simulink library "Enrg_conv_El_to_Mec_zfCetrax"  (R2016a)
settings: Solver=ode1  StartTime=0.0  StopTime=Inf  FixedStep=0.001  RelTol=1e-3
undefined symbols (not defined in the file): drvEmot_RefTqeMOT, FirstDrivenAxle_FirstDrivenAxleNoOfEmot, FirstDrivenAxleNoOfEmot, FMIKit, mec_fRollCoeffOverall, mec_iDiffAxle, mec_massVehicle_kg, mec_rWheelDriven, RefTqeMOT, SecondDrivenAxle_SecondDrivenAxleNoOfEmot, SecondDrivenAxleNoOfEmot
libraries: simulink_extras x3, Enrg_conv_El_to_Mec_zfCetrax x3
(part 1 of 3)
settings Model: Creator=SAHOPRA  LastModifiedBy=KGNANPR
settings DataIOCC: LimitDataPoints=on  SaveFormat=Array
settings OptimizationCC: BlockReduction=off  OptimizeBlockIOStorage=off  BufferReuse=off  GlobalBufferReuse=off  ExpressionFolding=off  ExpressionDepthLimit=2147483647  LocalBlockOutputs=off
settings DebuggingCC: UnderspecifiedInitializationDetection=Classic  MergeDetectMultiDrivingBlocksExec=none  SolverPrmCheckMsg=warning  StateNameClashWarn=warning
settings HardwareCC: ProdBitPerPointer=32  ProdLargestAtomicFloat=None  ProdIntDivRoundTo=Undefined  ProdEndianess=Unspecified  ProdWordSize=32  ProdHWDeviceType=32-bit Generic
settings ModelReferenceCC: PropagateSignalLabelsOutOfModel=off
settings SFSimCC: SimUserSources="\"C:\\ORNOVNU\\01_DIVe\\drl_dev_hvlv_work\\ldDevProj\\case\\c000\\Content\\phys\\hvs\\Support\\FMIToolkit\\FMIKit-Simulink-2.9\\src\\FMU.cpp\" \"C:\\ORNOVNU\\01_DIVe\\drl_dev_hvlv_work\\ldDevProj\\case\\c000\\Content\\phys\\hvs\\Support\\FMIToolkit\\FMIKit-Simulink-2.9\\src\\FMU1.cpp\" \"C:\\ORNOVNU\\01_DIVe\\drl_dev_hvlv_work\\ldDevProj\\case\\c000\\Content\\phys\\hvs\\Support\\FMIToolkit\\FMIKit-Simulink-2.9\\src\\FMU2.cpp\" \"C:\\ORNOVNU\\01_DIVe\\drm_dev_hvlv_work\\Content\\phys\\hvs\\Support\\FMIToolkit\\FMIKit-Simulink-2.9\\src\\FMU.cpp\" \"C:\\ORNOVNU\\01_DIVe\\drm_dev_hvlv_work\\Content\\phys\\hvs\\Support\\FMIToolkit\\FMIKit-Simulink-2.9\\src\\FMU1.cpp\" \"C:\\ORNOVNU\\01_DIVe\\drm_dev_hvlv_work\\Content\\phys\\hvs\\Support\\FMIToolkit\\FMIKit-Simulink-2.9\\src\\FMU2.cpp\" \"C:\\ORNOVNU\\01_DIVe\\drm_dev_hvlv_work\\Content\\phys\\hvs\\detailed\\Support\\FMIToolkit\\FMIKit-Simulink-2.9\\src\\FMU.cpp\" \"C:\\ORNOVNU\\01_DIVe\\drm_dev_hvlv_work\\Content\\phys\\hvs\\detailed\\Support\\FMIToolkit\\FMIKit-Simulink-2.9\\src\\FMU1.cpp\" \"C:\\ORNOVNU\\01_DIVe\\drm_dev_hvlv_work\\Content\\phys\\hvs\\detailed\\Support\\FMIToolkit\\FMIKit-Simulink-2.9\\src\\FMU2.cpp\" \"Y:\\03_Tasks\\20210223_OrNu_HVSDive_BoschModelle\\02_WIP\\FMIKit-Simulink-2.9\\src\\FMU.cpp\" \"Y:\\03_Tasks\\20210223_OrNu_HVSDive_BoschModelle\\02_WIP\\FMIKit-Simulink-2.9\\src\\FMU1.cpp\" \"Y:\\03_Tasks\\20210223_OrNu_HVSDive_BoschModelle\\02_WIP\\FMIKit-Simulink-2.9\\src\\FMU2.cpp\" \"C:\\Temp_Data\\eBus_work\\Content\\phys\\hvs\\detailed\\Support\\FMIToolkit\\FMIKit-Simulink-2.9\\src\\FMU.cpp\" \"C:\\Temp_Data\\eBus_work\\Content\\phys\\hvs\\detailed\\Support\\FMIToolkit\\FMIKit-Simulink-2.9\\src\\FMU1.cpp\" \"C:\\Temp_Data\\eBus_work\\Content\\phys\\hvs\\detailed\\Support\\FMIToolkit\\FMIKit-Simulink-2.9\\src\\FMU2.cpp\" \"C:\\Temp_Data\\DIVeMB\\00_eBus_Work\\Content\\phys\\hvs\\detailed\\Support\\FMIToolkit\\FMIKit-Simulink-2.9\\src\\FMU.cpp\" \"C:\\Temp_Data\\DIVeMB\\00_eBus_Work\\Content\\phys\\hvs\\detailed\\Support\\FMIToolkit\\FMIKit-Simulink-2.9\\src\\FMU1.cpp\" \"C:\\Temp_Data\\DIVeMB\\00_eBus_Work\\Content\\phys\\hvs\\detailed\\Support\\FMIToolkit\\FMIKit-Simulink-2.9\\src\\FMU2.cpp\" \"C:\\Temp_Data\\DIVeMB\\eBus_work\\Content\\phys\\hvs\\detailed\\Support\\FMIToolkit\\FMIKit-Simulink-2.9\\src\\FMU.cpp\" \"C:\\Temp_Data\\DIVeMB\\eBus_work\\Content\\phys\\hvs\\detailed\\Support\\FMIToolkit\\FMIKit-Simulink-2.9\\src\\FMU1.cpp\" \"C:\\Temp_Data\\DIVeMB\\eBus_work\\Content\\phys\\hvs\\detailed\\Support\\FMIToolkit\\FMIKit-Simulink-2.9\\src\\FMU2.cpp\""  SimUserIncludeDirs="\"C:\\ORNOVNU\\01_DIVe\\drl_dev_hvlv_work\\ldDevProj\\case\\c000\\Content\\phys\\hvs\\Support\\FMIToolkit\\FMIKit-Simulink-2.9\\include\" \"C:\\ORNOVNU\\01_DIVe\\drm_dev_hvlv_work\\Content\\phys\\hvs\\Support\\FMIToolkit\\FMIKit-Simulink-2.9\\include\" \"C:\\ORNOVNU\\01_DIVe\\drm_dev_hvlv_work\\Content\\phys\\hvs\\detailed\\Support\\FMIToolkit\\FMIKit-Simulink-2.9\\include\" \"Y:\\03_Tasks\\20210223_OrNu_HVSDive_BoschModelle\\02_WIP\\FMIKit-Simulink-2.9\\include\" \"C:\\Temp_Data\\eBus_work\\Content\\phys\\hvs\\detailed\\Support\\FMIToolkit\\FMIKit-Simulink-2.9\\include\" \"C:\\Temp_Data\\DIVeMB\\00_eBus_Work\\Content\\phys\\hvs\\detailed\\Support\\FMIToolkit\\FMIKit-Simulink-2.9\\include\" \"C:\\Temp_Data\\DIVeMB\\eBus_work\\Content\\phys\\hvs\\detailed\\Support\\FMIToolkit\\FMIKit-Simulink-2.9\\include\""
settings RTWCC: SystemTargetFile=rti1005.tlc  MakeCommand=make_rti  TemplateMakefile=rti1005.tmf  Description=dSPACE DS1005 Hardware Platform  CustomInclude="\"C:\\ORNOVNU\\01_DIVe\\drl_dev_hvlv_work\\ldDevProj\\case\\c000\\Content\\phys\\hvs\\Support\\FMIToolkit\\FMIKit-Simulink-2.9\\include\" \"C:\\ORNOVNU\\01_DIVe\\drm_dev_hvlv_work\\Content\\phys\\hvs\\Support\\FMIToolkit\\FMIKit-Simulink-2.9\\include\" \"C:\\ORNOVNU\\01_DIVe\\drm_dev_hvlv_work\\Content\\phys\\hvs\\detailed\\Support\\FMIToolkit\\FMIKit-Simulink-2.9\\include\" \"Y:\\03_Tasks\\20210223_OrNu_HVSDive_BoschModelle\\02_WIP\\FMIKit-Simulink-2.9\\include\" \"C:\\Temp_Data\\eBus_work\\Content\\phys\\hvs\\detailed\\Support\\FMIToolkit\\FMIKit-Simulink-2.9\\include\" \"C:\\Temp_Data\\DIVeMB\\00_eBus_Work\\Content\\phys\\hvs\\detailed\\Support\\FMIToolkit\\FMIKit-Simulink-2.9\\include\" \"C:\\Temp_Data\\DIVeMB\\eBus_work\\Content\\phys\\hvs\\detailed\\Support\\FMIToolkit\\FMIKit-Simulink-2.9\\include\""  CustomSource="\"C:\\ORNOVNU\\01_DIVe\\drl_dev_hvlv_work\\ldDevProj\\case\\c000\\Content\\phys\\hvs\\Support\\FMIToolkit\\FMIKit-Simulink-2.9\\src\\FMU.cpp\" \"C:\\ORNOVNU\\01_DIVe\\drl_dev_hvlv_work\\ldDevProj\\case\\c000\\Content\\phys\\hvs\\Support\\FMIToolkit\\FMIKit-Simulink-2.9\\src\\FMU1.cpp\" \"C:\\ORNOVNU\\01_DIVe\\drl_dev_hvlv_work\\ldDevProj\\case\\c000\\Content\\phys\\hvs\\Support\\FMIToolkit\\FMIKit-Simulink-2.9\\src\\FMU2.cpp\" \"C:\\ORNOVNU\\01_DIVe\\drm_dev_hvlv_work\\Content\\phys\\hvs\\Support\\FMIToolkit\\FMIKit-Simulink-2.9\\src\\FMU.cpp\" \"C:\\ORNOVNU\\01_DIVe\\drm_dev_hvlv_work\\Content\\phys\\hvs\\Support\\FMIToolkit\\FMIKit-Simulink-2.9\\src\\FMU1.cpp\" \"C:\\ORNOVNU\\01_DIVe\\drm_dev_hvlv_work\\Content\\phys\\hvs\\Support\\FMIToolkit\\FMIKit-Simulink-2.9\\src\\FMU2.cpp\" \"C:\\ORNOVNU\\01_DIVe\\drm_dev_hvlv_work\\Content\\phys\\hvs\\detailed\\Support\\FMIToolkit\\FMIKit-Simulink-2.9\\src\\FMU.cpp\" \"C:\\ORNOVNU\\01_DIVe\\drm_dev_hvlv_work\\Content\\phys\\hvs\\detailed\\Support\\FMIToolkit\\FMIKit-Simulink-2.9\\src\\FMU1.cpp\" \"C:\\ORNOVNU\\01_DIVe\\drm_dev_hvlv_work\\Content\\phys\\hvs\\detailed\\Support\\FMIToolkit\\FMIKit-Simulink-2.9\\src\\FMU2.cpp\" \"Y:\\03_Tasks\\20210223_OrNu_HVSDive_BoschModelle\\02_WIP\\FMIKit-Simulink-2.9\\src\\FMU.cpp\" \"Y:\\03_Tasks\\20210223_OrNu_HVSDive_BoschModelle\\02_WIP\\FMIKit-Simulink-2.9\\src\\FMU1.cpp\" \"Y:\\03_Tasks\\20210223_OrNu_HVSDive_BoschModelle\\02_WIP\\FMIKit-Simulink-2.9\\src\\FMU2.cpp\" \"C:\\Temp_Data\\eBus_work\\Content\\phys\\hvs\\detailed\\Support\\FMIToolkit\\FMIKit-Simulink-2.9\\src\\FMU.cpp\" \"C:\\Temp_Data\\eBus_work\\Content\\phys\\hvs\\detailed\\Support\\FMIToolkit\\FMIKit-Simulink-2.9\\src\\FMU1.cpp\" \"C:\\Temp_Data\\eBus_work\\Content\\phys\\hvs\\detailed\\Support\\FMIToolkit\\FMIKit-Simulink-2.9\\src\\FMU2.cpp\" \"C:\\Temp_Data\\DIVeMB\\00_eBus_Work\\Content\\phys\\hvs\\detailed\\Support\\FMIToolkit\\FMIKit-Simulink-2.9\\src\\FMU.cpp\" \"C:\\Temp_Data\\DIVeMB\\00_eBus_Work\\Content\\phys\\hvs\\detailed\\Support\\FMIToolkit\\FMIKit-Simulink-2.9\\src\\FMU1.cpp\" \"C:\\Temp_Data\\DIVeMB\\00_eBus_Work\\Content\\phys\\hvs\\detailed\\Support\\FMIToolkit\\FMIKit-Simulink-2.9\\src\\FMU2.cpp\" \"C:\\Temp_Data\\DIVeMB\\eBus_work\\Content\\phys\\hvs\\detailed\\Support\\FMIToolkit\\FMIKit-Simulink-2.9\\src\\FMU.cpp\" \"C:\\Temp_Data\\DIVeMB\\eBus_work\\Content\\phys\\hvs\\detailed\\Support\\FMIToolkit\\FMIKit-Simulink-2.9\\src\\FMU1.cpp\" \"C:\\Temp_Data\\DIVeMB\\eBus_work\\Content\\phys\\hvs\\detailed\\Support\\FMIToolkit\\FMIKit-Simulink-2.9\\src\\FMU2.cpp\""
settings STFCustomTargetCC: ModelReferenceCompliant=off  GeneratePreprocessorConditionals=Disable all  CombineOutputUpdateFcns=on  MatFileLogging=on  CPPClassGenCompliant=on  GRTInterface=off  SystemTargetFile=rti1005.tlc
settings GRTTargetCC: ModelReferenceCompliant=off  ParMdlRefBuildCompliant=off  CompOptLevelCompliant=off  ConcurrentExecutionCompliant=off  UseToolchainInfoCompliant=off
settings ConfigComp: CovModelRefEnable=Off

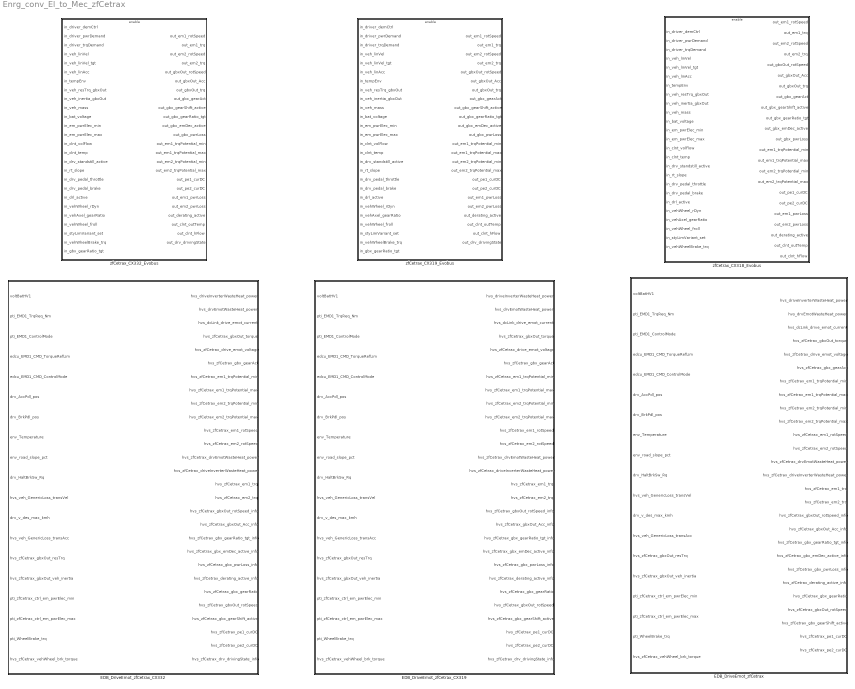
== system Enrg_conv_El_to_Mec_zfCetrax ==
  EDB_DriveEmot_zfCetrax : Subsystem
  EDB_DriveEmot_zfCetrax_CX319 : Subsystem
  EDB_DriveEmot_zfCetrax_CX332 : Subsystem
  zfCetrax_CX318_Evobus : Subsystem  mask(MapModule){}
  zfCetrax_CX319_Evobus : Subsystem  mask(MapModule){}
  zfCetrax_CX332_Evobus : Subsystem  mask(MapModule){}

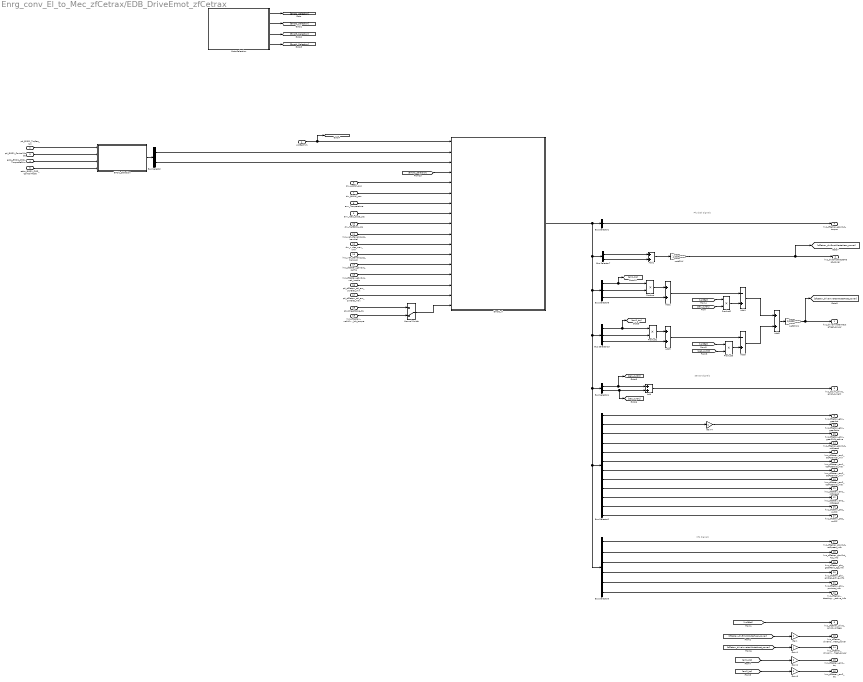
== system Enrg_conv_El_to_Mec_zfCetrax/EDB_DriveEmot_zfCetrax ==
  note: Physical Signals
  note: Sensor Signals
  note: Info Signals
  voltBatHV1 : Inport
  pti_EMD1_TrqReq_Nm : Inport  Port=2
  pti_EMD1_ControlMode : Inport  Port=3
  edcu_EMD1_CMD_TorqueRefLim : Inport  Port=4
  edcu_EMD1_CMD_ControlMode : Inport  Port=5
  drv_AccPdl_pos : Inport  Port=6
  drv_BrkPdl_pos : Inport  Port=7
  env_Temperature : Inport  Port=8
  env_road_slope_pct : Inport  Port=9
  drv_HaltBrkSw_Rq : Inport  Port=10
  hvs_veh_GenericLoss_transVel : Inport  Port=11
  drv_v_des_max_kmh : Inport  Port=12
  hvs_veh_GenericLoss_transAcc : Inport  Port=13
  hvs_zfCetrax_gbxOut_resTrq : Inport  Port=14
  hvs_zfCetrax_gbxOut_veh_inertia : Inport  Port=15
  pti_zfCetrax_ctrl_em_pwrElec_min : Inport  Port=16
  pti_zfCetrax_ctrl_em_pwrElec_max : Inport  Port=17
  pti_WheelBrake_trq : Inport  Port=18
  hvs_zfCetrax_vehWheel_brk_torque : Inport  Port=19
  Add{,1..3,6} (5 alike) : Sum
  Add4 : Sum  Inputs=-+
  Add5 : Sum  Inputs=-+
  Bus Selector : BusSelector  OutputSignals=EMD1_TrqReq_Nm,EMD1_ControlMode
  Bus Selector1 : BusSelector  OutputSignals=gbx_out.gbxOut_trq
  Bus Selector13 : BusSelector  OutputSignals=em2_out.em2_trq,em2_out.em2_rotSpeed,em2_out.em2_pwrLoss
  Bus Selector2 : BusSelector  OutputSignals=gbx_out.gbx_gearAct,gbx_out.gbx_gearRatio_tgt,gbx_out.gbx_gearShift_active,gbx_out.gbxOut_rotSpeed,em1_out.em1_trqPotential_min,em1_out.em1_trqPotential_max,em2_out.em2_trqPotential_min,em2_out.em2_trqPotential_max,em1_out.em1_rotSpeed,em2_out.em2_rotSpeed,em1_out.pe1_curDC,em2_out.pe2_curDC
  Bus Selector3 : BusSelector  OutputSignals=gbx_out.gbxOut_rotSpeed,gbx_out.gbxOut_Acc,gbx_out.gbx_gearRatio_tgt,gbx_out.gbx_emDec_active,gbx_out.gbx_pwrLoss,gbx_out.derating_active
  Bus Selector4 : BusSelector  OutputSignals=em1_out.pe1_curDC,em2_out.pe2_curDC
  Bus Selector7 : BusSelector  OutputSignals=em1_out.em1_pwrLoss,em2_out.em2_pwrLoss
  Bus Selector8 : BusSelector  OutputSignals=em1_out.em1_trq,em1_out.em1_rotSpeed,em1_out.em1_pwrLoss
  EMD1_Selection : Subsystem
  Emot1_4 : Subsystem
  Gain{,1..4} (5 alike) : Gain
  Manual Switch : ManualSwitch  CurrentSetting=0
  MotorSelection : Subsystem
  Product{,1..3} (4 alike) : Product
  watt2kW : Gain  Gain=1/1000
  watt2kW1 : Gain  Gain=1/1000
  hvs_driveInverterWasteHeat_power : Outport
  hvs_drvEmotWasteHeat_power : Outport  Port=2
  hvs_dcLink_drive_emot_current : Outport  Port=3
  hvs_zfCetrax_gbxOut_torque : Outport  Port=4
  hvs_zfCetrax_drive_emot_voltage : Outport  Port=5
  hvs_zfCetrax_gbx_gearAct : Outport  Port=6
  hvs_zfCetrax_em1_trqPotential_min : Outport  Port=7
  hvs_zfCetrax_em1_trqPotential_max : Outport  Port=8
  hvs_zfCetrax_em2_trqPotential_min : Outport  Port=9
  hvs_zfCetrax_em2_trqPotential_max : Outport  Port=10
  hvs_zfCetrax_em1_rotSpeed : Outport  Port=11
  hvs_zfCetrax_em2_rotSpeed : Outport  Port=12
  hvs_zfCetrax_drvEmotWasteHeat_power : Outport  Port=13
  hvs_zfCetrax_driveInverterWasteHeat_power : Outport  Port=14
  hvs_zfCetrax_em1_trq : Outport  Port=15
  hvs_zfCetrax_em2_trq : Outport  Port=16
  hvs_zfCetrax_gbxOut_rotSpeed_info : Outport  Port=17
  hvs_zfCetrax_gbxOut_Acc_info : Outport  Port=18
  hvs_zfCetrax_gbx_gearRatio_tgt_info : Outport  Port=19
  hvs_zfCetrax_gbx_emDec_active_info : Outport  Port=20
  hvs_zfCetrax_gbx_pwrLoss_info : Outport  Port=21
  hvs_zfCetrax_derating_active_info : Outport  Port=22
  hvs_zfCetrax_gbx_gearRatio : Outport  Port=23
  hvs_zfCetrax_gbxOut_rotSpeed : Outport  Port=24
  hvs_zfCetrax_gbx_gearShift_active : Outport  Port=25
  hvs_zfCetrax_pe1_curDC : Outport  Port=26
  hvs_zfCetrax_pe2_curDC : Outport  Port=27
  wires:
  MotorSelection/1(Emot1_Selection) -> [Emot1_Selection]
  MotorSelection/2(Emot2_Selection) -> [Emot2_Selection]
  MotorSelection/3(Emot3_Selection) -> [Emot3_Selection]
  MotorSelection/4(Emot4_Selection) -> [Emot4_Selection]
  [Emot1_Selection] -> Emot1_4/4(Emot1_Selection)
  voltBatHV1/1 -> [voltBat], Emot1_4/1(voltBatHV1)
  pti_EMD1_TrqReq_Nm/1 -> EMD1_Selection/1(pti_EMD1_TrqReq_Nm)
  pti_EMD1_ControlMode/1 -> EMD1_Selection/2(pti_EMD1_ControlMode)
  edcu_EMD1_CMD_TorqueRefLim/1 -> EMD1_Selection/3(edcu_EMD1_CMD_TorqueRefLim)
  edcu_EMD1_CMD_ControlMode/1 -> EMD1_Selection/4(edcu_EMD1_CMD_ControlMode)
  EMD1_Selection/1(Signal) -> Bus Selector/1
  Bus Selector/1 -> Emot1_4/2(trqEmotDesPhy1)  "<EMD1_TrqReq_Nm>"
  Bus Selector/2 -> Emot1_4/3(emot_CMD1)  "<EMD1_ControlMode>"
  drv_AccPdl_pos/1 -> Emot1_4/5(drv_AccPdl_pos)
  drv_BrkPdl_pos/1 -> Emot1_4/6(drv_BrkPdl_pos)
  env_Temperature/1 -> Emot1_4/7(env_Temperature)
  env_road_slope_pct/1 -> Emot1_4/8(env_road_slope_pct)
  drv_HaltBrkSw_Rq/1 -> Emot1_4/9(drv_HaltBrkSw_Rq)
  hvs_veh_GenericLoss_transVel/1 -> Emot1_4/10(veh_linVel)
  pti_zfCetrax_ctrl_em_pwrElec_min/1 -> Emot1_4/15(em_pwrElec_min)
  drv_v_des_max_kmh/1 -> Emot1_4/11(veh_linVel_tgt)
  hvs_veh_GenericLoss_transAcc/1 -> Emot1_4/12(veh_linAcc)
  pti_zfCetrax_ctrl_em_pwrElec_max/1 -> Emot1_4/16(em_pwrElec_max)
  hvs_zfCetrax_gbxOut_resTrq/1 -> Emot1_4/13(veh_resTrq_gbxOut)
  hvs_zfCetrax_gbxOut_veh_inertia/1 -> Emot1_4/14(veh_inertial_gbxOut)
  Emot1_4/1(ceTrax) -> Bus Selector4/1, Bus Selector3/1, Bus Selector2/1, Bus Selector13/1, Bus Selector8/1, Bus Selector7/1, Bus Selector1/1
  Bus Selector1/1 -> hvs_zfCetrax_gbxOut_torque/1  "<gbxOut_trq>"
  Bus Selector4/1 -> Add/1, [pe1_curDC]  "<pe1_curDC>"
  Bus Selector4/2 -> [pe2_curDC], Add/2  "<pe2_curDC>"
  Add/1 -> hvs_dcLink_drive_emot_current/1
  Bus Selector7/1 -> Add1/1  "<em1_pwrLoss>"
  Bus Selector7/2 -> Add1/2  "<em2_pwrLoss>"
  Add1/1 -> watt2kW/1
  Bus Selector8/2 -> Product/2  "<em1_rotSpeed>"
  Bus Selector8/1 -> [em1_trq], Product/1  "<em1_trq>"
  Product/1 -> Add2/1
  Bus Selector8/3 -> Add2/2  "<em1_pwrLoss>"
  Add2/1 -> Add4/1
  Bus Selector13/1 -> [em2_trq], Product1/1  "<em2_trq>"
  Bus Selector13/2 -> Product1/2  "<em2_rotSpeed>"
  Product1/1 -> Add3/1
  Bus Selector13/3 -> Add3/2  "<em2_pwrLoss>"
  Add3/1 -> Add5/1
  [pe1_curDC] -> Product2/2
  Product2/1 -> Add4/2
  [voltBat] -> Product2/1
  [pe2_curDC] -> Product3/2
  Product3/1 -> Add5/2
  [voltBat] -> Product3/1
  Add4/1 -> Add6/1
  Add5/1 -> Add6/2
  Add6/1 -> watt2kW1/1
  watt2kW/1 -> hvs_drvEmotWasteHeat_power/1, [zfCetrax_drvEmotWasteHear_power]
  watt2kW1/1 -> hvs_driveInverterWasteHeat_power/1, [zfCetrax_driveInverterWasteHeat_power]
  [voltBat] -> hvs_zfCetrax_drive_emot_voltage/1
  Bus Selector2/1 -> hvs_zfCetrax_gbx_gearAct/1  "<gbx_gearAct>"
  Bus Selector2/5 -> hvs_zfCetrax_em1_trqPotential_min/1  "<em1_trqPotential_min>"
  Bus Selector2/6 -> hvs_zfCetrax_em1_trqPotential_max/1  "<em1_trqPotential_max>"
  Bus Selector2/7 -> hvs_zfCetrax_em2_trqPotential_min/1  "<em2_trqPotential_min>"
  Bus Selector2/8 -> hvs_zfCetrax_em2_trqPotential_max/1  "<em2_trqPotential_max>"
  Bus Selector2/10 -> hvs_zfCetrax_em2_rotSpeed/1  "<em2_rotSpeed>"
  Bus Selector2/9 -> hvs_zfCetrax_em1_rotSpeed/1  "<em1_rotSpeed>"
  [zfCetrax_drvEmotWasteHear_power] -> Gain/1
  Gain/1 -> hvs_zfCetrax_drvEmotWasteHeat_power/1
  [zfCetrax_driveInverterWasteHeat_power] -> Gain1/1
  Gain1/1 -> hvs_zfCetrax_driveInverterWasteHeat_power/1
  [em1_trq] -> Gain2/1
  [em2_trq] -> Gain3/1
  Gain2/1 -> hvs_zfCetrax_em1_trq/1
  Gain3/1 -> hvs_zfCetrax_em2_trq/1
  pti_WheelBrake_trq/1 -> Manual Switch/1
  Bus Selector3/1 -> hvs_zfCetrax_gbxOut_rotSpeed_info/1  "<gbxOut_rotSpeed>"
  Bus Selector3/2 -> hvs_zfCetrax_gbxOut_Acc_info/1  "<gbxOut_Acc>"
  Bus Selector3/3 -> hvs_zfCetrax_gbx_gearRatio_tgt_info/1  "<gbx_gearRatio_tgt>"
  Bus Selector3/4 -> hvs_zfCetrax_gbx_emDec_active_info/1  "<gbx_emDec_active>"
  Bus Selector3/5 -> hvs_zfCetrax_gbx_pwrLoss_info/1  "<gbx_pwrLoss>"
  Bus Selector3/6 -> hvs_zfCetrax_derating_active_info/1  "<derating_active>"
  Bus Selector2/2 -> Gain4/1  "<gbx_gearRatio_tgt>"
  Gain4/1 -> hvs_zfCetrax_gbx_gearRatio/1
  hvs_zfCetrax_vehWheel_brk_torque/1 -> Manual Switch/2
  Manual Switch/1 -> Emot1_4/17(pti_WheelBrake_trq)
  Bus Selector2/4 -> hvs_zfCetrax_gbxOut_rotSpeed/1  "<gbxOut_rotSpeed>"
  Bus Selector2/3 -> hvs_zfCetrax_gbx_gearShift_active/1  "<gbx_gearShift_active>"
  Bus Selector2/11 -> hvs_zfCetrax_pe1_curDC/1  "<pe1_curDC>"
  Bus Selector2/12 -> hvs_zfCetrax_pe2_curDC/1  "<pe2_curDC>"

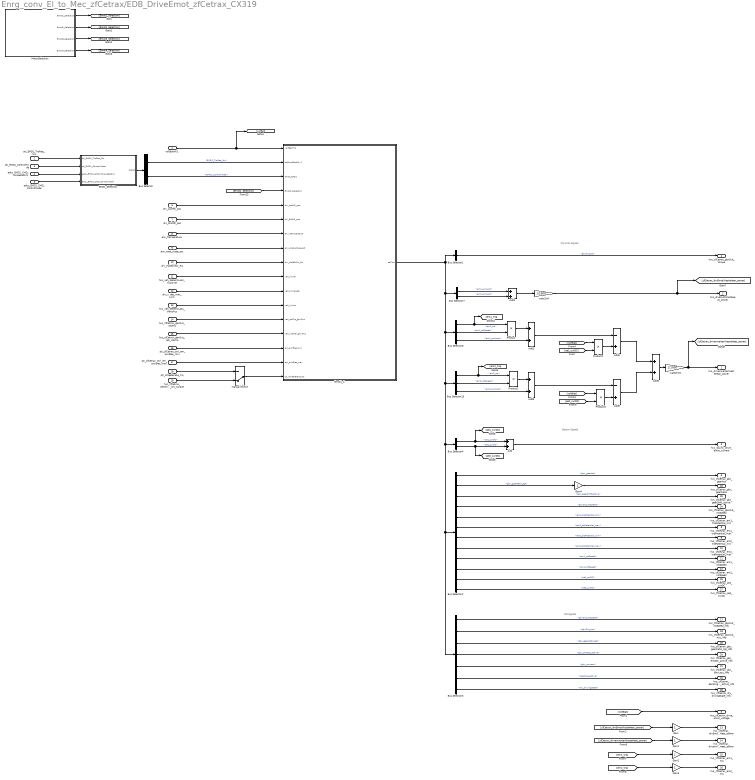
== system Enrg_conv_El_to_Mec_zfCetrax/EDB_DriveEmot_zfCetrax_CX319 ==
  note: Info Signals
  note: Sensor Signals
  note: Physical Signals
  voltBatHV1 : Inport
  pti_EMD1_TrqReq_Nm : Inport  Port=2
  pti_EMD1_ControlMode : Inport  Port=3
  edcu_EMD1_CMD_TorqueRefLim : Inport  Port=4
  edcu_EMD1_CMD_ControlMode : Inport  Port=5
  drv_AccPdl_pos : Inport  Port=6
  drv_BrkPdl_pos : Inport  Port=7
  env_Temperature : Inport  Port=8
  env_road_slope_pct : Inport  Port=9
  drv_HaltBrkSw_Rq : Inport  Port=10
  hvs_veh_GenericLoss_transVel : Inport  Port=11
  drv_v_des_max_kmh : Inport  Port=12
  hvs_veh_GenericLoss_transAcc : Inport  Port=13
  hvs_zfCetrax_gbxOut_resTrq : Inport  Port=14
  hvs_zfCetrax_gbxOut_veh_inertia : Inport  Port=15
  pti_zfCetrax_ctrl_em_pwrElec_min : Inport  Port=16
  pti_zfCetrax_ctrl_em_pwrElec_max : Inport  Port=17
  pti_WheelBrake_trq : Inport  Port=18
  hvs_zfCetrax_vehWheel_brk_torque : Inport  Port=19
  Add{,1..3,6} (5 alike) : Sum
  Add4 : Sum  Inputs=-+
  Add5 : Sum  Inputs=-+
  Bus Selector : BusSelector  OutputSignals=EMD1_TrqReq_Nm,EMD1_ControlMode
  Bus Selector1 : BusSelector  OutputSignals=gbx_out.gbxOut_trq
  Bus Selector13 : BusSelector  OutputSignals=em2_out.em2_trq,em2_out.em2_rotSpeed,em2_out.em2_pwrLoss
  Bus Selector2 : BusSelector  OutputSignals=gbx_out.gbx_gearAct,gbx_out.gbx_gearRatio_tgt,gbx_out.gbx_gearShift_active,gbx_out.gbxOut_rotSpeed,em1_out.em1_trqPotential_min,em1_out.em1_trqPotential_max,em2_out.em2_trqPotential_min,em2_out.em2_trqPotential_max,em1_out.em1_rotSpeed,em2_out.em2_rotSpeed,em1_out.pe1_curDC,em2_out.pe2_curDC
  Bus Selector3 : BusSelector  OutputSignals=gbx_out.gbxOut_rotSpeed,gbx_out.gbxOut_Acc,gbx_out.gbx_gearRatio_tgt,gbx_out.gbx_emDec_active,gbx_out.gbx_pwrLoss,gbx_out.derating_active,gbx_out.drv_drivingState
  Bus Selector4 : BusSelector  OutputSignals=em1_out.pe1_curDC,em2_out.pe2_curDC
  Bus Selector7 : BusSelector  OutputSignals=em1_out.em1_pwrLoss,em2_out.em2_pwrLoss
  Bus Selector8 : BusSelector  OutputSignals=em1_out.em1_trq,em1_out.em1_rotSpeed,em1_out.em1_pwrLoss
  EMD1_Selection : Subsystem
  Emot1_4 : Subsystem
  Gain{,1..4} (5 alike) : Gain
  Manual Switch : ManualSwitch  CurrentSetting=0
  MotorSelection : Subsystem
  Product{,1..3} (4 alike) : Product
  watt2kW : Gain  Gain=1/1000
  watt2kW1 : Gain  Gain=1/1000
  hvs_driveInverterWasteHeat_power : Outport
  hvs_drvEmotWasteHeat_power : Outport  Port=2
  hvs_dcLink_drive_emot_current : Outport  Port=3
  hvs_zfCetrax_gbxOut_torque : Outport  Port=4
  hvs_zfCetrax_drive_emot_voltage : Outport  Port=5
  hvs_zfCetrax_gbx_gearAct : Outport  Port=6
  hvs_zfCetrax_em1_trqPotential_min : Outport  Port=7
  hvs_zfCetrax_em1_trqPotential_max : Outport  Port=8
  hvs_zfCetrax_em2_trqPotential_min : Outport  Port=9
  hvs_zfCetrax_em2_trqPotential_max : Outport  Port=10
  hvs_zfCetrax_em1_rotSpeed : Outport  Port=11
  hvs_zfCetrax_em2_rotSpeed : Outport  Port=12
  hvs_zfCetrax_drvEmotWasteHeat_power : Outport  Port=13
  hvs_zfCetrax_driveInverterWasteHeat_power : Outport  Port=14
  hvs_zfCetrax_em1_trq : Outport  Port=15
  hvs_zfCetrax_em2_trq : Outport  Port=16
  hvs_zfCetrax_gbxOut_rotSpeed_info : Outport  Port=17
  hvs_zfCetrax_gbxOut_Acc_info : Outport  Port=18
  hvs_zfCetrax_gbx_gearRatio_tgt_info : Outport  Port=19
  hvs_zfCetrax_gbx_emDec_active_info : Outport  Port=20
  hvs_zfCetrax_gbx_pwrLoss_info : Outport  Port=21
  hvs_zfCetrax_derating_active_info : Outport  Port=22
  hvs_zfCetrax_gbx_gearRatio : Outport  Port=23
  hvs_zfCetrax_gbxOut_rotSpeed : Outport  Port=24
  hvs_zfCetrax_gbx_gearShift_active : Outport  Port=25
  hvs_zfCetrax_pe1_curDC : Outport  Port=26
  hvs_zfCetrax_pe2_curDC : Outport  Port=27
  hvs_zfCetrax_drv_drivingState_info : Outport  Port=28
  wires:
  Bus Selector3/7 -> hvs_zfCetrax_drv_drivingState_info/1  "<drv_drivingState>"
  Bus Selector2/12 -> hvs_zfCetrax_pe2_curDC/1  "<pe2_curDC>"
  Bus Selector2/11 -> hvs_zfCetrax_pe1_curDC/1  "<pe1_curDC>"
  Bus Selector2/3 -> hvs_zfCetrax_gbx_gearShift_active/1  "<gbx_gearShift_active>"
  Bus Selector2/4 -> hvs_zfCetrax_gbxOut_rotSpeed/1  "<gbxOut_rotSpeed>"
  Manual Switch/1 -> Emot1_4/17(pti_WheelBrake_trq)
  hvs_zfCetrax_vehWheel_brk_torque/1 -> Manual Switch/2
  Gain4/1 -> hvs_zfCetrax_gbx_gearRatio/1
  Bus Selector2/2 -> Gain4/1  "<gbx_gearRatio_tgt>"
  Bus Selector3/6 -> hvs_zfCetrax_derating_active_info/1  "<derating_active>"
  Bus Selector3/5 -> hvs_zfCetrax_gbx_pwrLoss_info/1  "<gbx_pwrLoss>"
  Bus Selector3/4 -> hvs_zfCetrax_gbx_emDec_active_info/1  "<gbx_emDec_active>"
  Bus Selector3/3 -> hvs_zfCetrax_gbx_gearRatio_tgt_info/1  "<gbx_gearRatio_tgt>"
  Bus Selector3/2 -> hvs_zfCetrax_gbxOut_Acc_info/1  "<gbxOut_Acc>"
  Bus Selector3/1 -> hvs_zfCetrax_gbxOut_rotSpeed_info/1  "<gbxOut_rotSpeed>"
  pti_WheelBrake_trq/1 -> Manual Switch/1
  Gain3/1 -> hvs_zfCetrax_em2_trq/1
  Gain2/1 -> hvs_zfCetrax_em1_trq/1
  [em2_trq] -> Gain3/1
  [em1_trq] -> Gain2/1
  Gain1/1 -> hvs_zfCetrax_driveInverterWasteHeat_power/1
  [zfCetrax_driveInverterWasteHeat_power] -> Gain1/1
  Gain/1 -> hvs_zfCetrax_drvEmotWasteHeat_power/1
  [zfCetrax_drvEmotWasteHear_power] -> Gain/1
  Bus Selector2/9 -> hvs_zfCetrax_em1_rotSpeed/1  "<em1_rotSpeed>"
  Bus Selector2/10 -> hvs_zfCetrax_em2_rotSpeed/1  "<em2_rotSpeed>"
  Bus Selector2/8 -> hvs_zfCetrax_em2_trqPotential_max/1  "<em2_trqPotential_max>"
  Bus Selector2/7 -> hvs_zfCetrax_em2_trqPotential_min/1  "<em2_trqPotential_min>"
  Bus Selector2/6 -> hvs_zfCetrax_em1_trqPotential_max/1  "<em1_trqPotential_max>"
  Bus Selector2/5 -> hvs_zfCetrax_em1_trqPotential_min/1  "<em1_trqPotential_min>"
  Bus Selector2/1 -> hvs_zfCetrax_gbx_gearAct/1  "<gbx_gearAct>"
  [voltBat] -> hvs_zfCetrax_drive_emot_voltage/1
  watt2kW1/1 -> [zfCetrax_driveInverterWasteHeat_power], hvs_driveInverterWasteHeat_power/1
  watt2kW/1 -> [zfCetrax_drvEmotWasteHear_power], hvs_drvEmotWasteHeat_power/1
  Add6/1 -> watt2kW1/1
  Add5/1 -> Add6/2
  Add4/1 -> Add6/1
  [voltBat] -> Product3/1
  Product3/1 -> Add5/2
  [pe2_curDC] -> Product3/2
  [voltBat] -> Product2/1
  Product2/1 -> Add4/2
  [pe1_curDC] -> Product2/2
  Add3/1 -> Add5/1
  Bus Selector13/3 -> Add3/2  "<em2_pwrLoss>"
  Product1/1 -> Add3/1
  Bus Selector13/2 -> Product1/2  "<em2_rotSpeed>"
  Bus Selector13/1 -> Product1/1, [em2_trq]  "<em2_trq>"
  Add2/1 -> Add4/1
  Bus Selector8/3 -> Add2/2  "<em1_pwrLoss>"
  Product/1 -> Add2/1
  Bus Selector8/1 -> Product/1, [em1_trq]  "<em1_trq>"
  Bus Selector8/2 -> Product/2  "<em1_rotSpeed>"
  Add1/1 -> watt2kW/1
  Bus Selector7/2 -> Add1/2  "<em2_pwrLoss>"
  Bus Selector7/1 -> Add1/1  "<em1_pwrLoss>"
  Add/1 -> hvs_dcLink_drive_emot_current/1
  Bus Selector4/2 -> Add/2, [pe2_curDC]  "<pe2_curDC>"
  Bus Selector4/1 -> [pe1_curDC], Add/1  "<pe1_curDC>"
  Bus Selector1/1 -> hvs_zfCetrax_gbxOut_torque/1  "<gbxOut_trq>"
  Emot1_4/1(ceTrax) -> Bus Selector1/1, Bus Selector7/1, Bus Selector8/1, Bus Selector13/1, Bus Selector2/1, Bus Selector3/1, Bus Selector4/1
  hvs_zfCetrax_gbxOut_veh_inertia/1 -> Emot1_4/14(veh_inertial_gbxOut)
  hvs_zfCetrax_gbxOut_resTrq/1 -> Emot1_4/13(veh_resTrq_gbxOut)
  pti_zfCetrax_ctrl_em_pwrElec_max/1 -> Emot1_4/16(em_pwrElec_max)
  hvs_veh_GenericLoss_transAcc/1 -> Emot1_4/12(veh_linAcc)
  drv_v_des_max_kmh/1 -> Emot1_4/11(veh_linVel_tgt)
  pti_zfCetrax_ctrl_em_pwrElec_min/1 -> Emot1_4/15(em_pwrElec_min)
  hvs_veh_GenericLoss_transVel/1 -> Emot1_4/10(veh_linVel)
  drv_HaltBrkSw_Rq/1 -> Emot1_4/9(drv_HaltBrkSw_Rq)
  env_road_slope_pct/1 -> Emot1_4/8(env_road_slope_pct)
  env_Temperature/1 -> Emot1_4/7(env_Temperature)
  drv_BrkPdl_pos/1 -> Emot1_4/6(drv_BrkPdl_pos)
  drv_AccPdl_pos/1 -> Emot1_4/5(drv_AccPdl_pos)
  Bus Selector/2 -> Emot1_4/3(emot_CMD1)  "<EMD1_ControlMode>"
  Bus Selector/1 -> Emot1_4/2(trqEmotDesPhy1)  "<EMD1_TrqReq_Nm>"
  EMD1_Selection/1(Signal) -> Bus Selector/1
  edcu_EMD1_CMD_ControlMode/1 -> EMD1_Selection/4(edcu_EMD1_CMD_ControlMode)
  edcu_EMD1_CMD_TorqueRefLim/1 -> EMD1_Selection/3(edcu_EMD1_CMD_TorqueRefLim)
  pti_EMD1_ControlMode/1 -> EMD1_Selection/2(pti_EMD1_ControlMode)
  pti_EMD1_TrqReq_Nm/1 -> EMD1_Selection/1(pti_EMD1_TrqReq_Nm)
  voltBatHV1/1 -> Emot1_4/1(voltBatHV1), [voltBat]
  [Emot1_Selection] -> Emot1_4/4(Emot1_Selection)
  MotorSelection/4(Emot4_Selection) -> [Emot4_Selection]
  MotorSelection/3(Emot3_Selection) -> [Emot3_Selection]
  MotorSelection/2(Emot2_Selection) -> [Emot2_Selection]
  MotorSelection/1(Emot1_Selection) -> [Emot1_Selection]

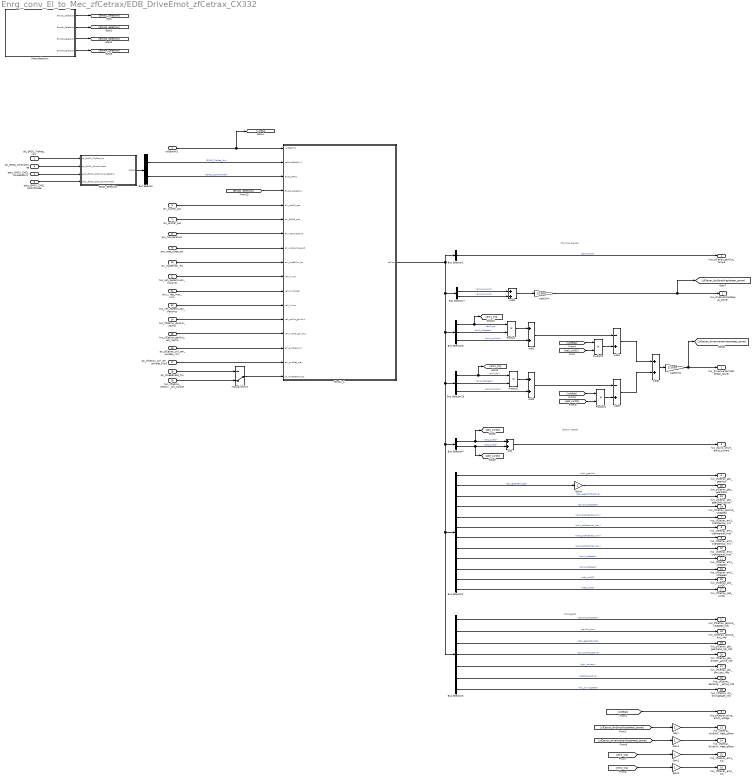
== system Enrg_conv_El_to_Mec_zfCetrax/EDB_DriveEmot_zfCetrax_CX332 ==
  note: Physical Signals
  note: Sensor Signals
  note: Info Signals
  voltBatHV1 : Inport
  pti_EMD1_TrqReq_Nm : Inport  Port=2
  pti_EMD1_ControlMode : Inport  Port=3
  edcu_EMD1_CMD_TorqueRefLim : Inport  Port=4
  edcu_EMD1_CMD_ControlMode : Inport  Port=5
  drv_AccPdl_pos : Inport  Port=6
  drv_BrkPdl_pos : Inport  Port=7
  env_Temperature : Inport  Port=8
  env_road_slope_pct : Inport  Port=9
  drv_HaltBrkSw_Rq : Inport  Port=10
  hvs_veh_GenericLoss_transVel : Inport  Port=11
  drv_v_des_max_kmh : Inport  Port=12
  hvs_veh_GenericLoss_transAcc : Inport  Port=13
  hvs_zfCetrax_gbxOut_resTrq : Inport  Port=14
  hvs_zfCetrax_gbxOut_veh_inertia : Inport  Port=15
  pti_zfCetrax_ctrl_em_pwrElec_min : Inport  Port=16
  pti_zfCetrax_ctrl_em_pwrElec_max : Inport  Port=17
  pti_WheelBrake_trq : Inport  Port=18
  hvs_zfCetrax_vehWheel_brk_torque : Inport  Port=19
  Add{,1..3,6} (5 alike) : Sum
  Add4 : Sum  Inputs=-+
  Add5 : Sum  Inputs=-+
  Bus Selector : BusSelector  OutputSignals=EMD1_TrqReq_Nm,EMD1_ControlMode
  Bus Selector1 : BusSelector  OutputSignals=gbx_out.gbxOut_trq
  Bus Selector13 : BusSelector  OutputSignals=em2_out.em2_trq,em2_out.em2_rotSpeed,em2_out.em2_pwrLoss
  Bus Selector2 : BusSelector  OutputSignals=gbx_out.gbx_gearAct,gbx_out.gbx_gearRatio_tgt,gbx_out.gbx_gearShift_active,gbx_out.gbxOut_rotSpeed,em1_out.em1_trqPotential_min,em1_out.em1_trqPotential_max,em2_out.em2_trqPotential_min,em2_out.em2_trqPotential_max,em1_out.em1_rotSpeed,em2_out.em2_rotSpeed,em1_out.pe1_curDC,em2_out.pe2_curDC
  Bus Selector3 : BusSelector  OutputSignals=gbx_out.gbxOut_rotSpeed,gbx_out.gbxOut_Acc,gbx_out.gbx_gearRatio_tgt,gbx_out.gbx_emDec_active,gbx_out.gbx_pwrLoss,gbx_out.derating_active,gbx_out.drv_drivingState
  Bus Selector4 : BusSelector  OutputSignals=em1_out.pe1_curDC,em2_out.pe2_curDC
  Bus Selector7 : BusSelector  OutputSignals=em1_out.em1_pwrLoss,em2_out.em2_pwrLoss
  Bus Selector8 : BusSelector  OutputSignals=em1_out.em1_trq,em1_out.em1_rotSpeed,em1_out.em1_pwrLoss
  EMD1_Selection : Subsystem
  Emot1_4 : Subsystem
  Gain{,1..4} (5 alike) : Gain
  Manual Switch : ManualSwitch  CurrentSetting=0
  MotorSelection : Subsystem
  Product{,1..3} (4 alike) : Product
  watt2kW : Gain  Gain=1/1000
  watt2kW1 : Gain  Gain=1/1000
  hvs_driveInverterWasteHeat_power : Outport
  hvs_drvEmotWasteHeat_power : Outport  Port=2
  hvs_dcLink_drive_emot_current : Outport  Port=3
  hvs_zfCetrax_gbxOut_torque : Outport  Port=4
  hvs_zfCetrax_drive_emot_voltage : Outport  Port=5
  hvs_zfCetrax_gbx_gearAct : Outport  Port=6
  hvs_zfCetrax_em1_trqPotential_min : Outport  Port=7
  hvs_zfCetrax_em1_trqPotential_max : Outport  Port=8
  hvs_zfCetrax_em2_trqPotential_min : Outport  Port=9
  hvs_zfCetrax_em2_trqPotential_max : Outport  Port=10
  hvs_zfCetrax_em1_rotSpeed : Outport  Port=11
  hvs_zfCetrax_em2_rotSpeed : Outport  Port=12
  hvs_zfCetrax_drvEmotWasteHeat_power : Outport  Port=13
  hvs_zfCetrax_driveInverterWasteHeat_power : Outport  Port=14
  hvs_zfCetrax_em1_trq : Outport  Port=15
  hvs_zfCetrax_em2_trq : Outport  Port=16
  hvs_zfCetrax_gbxOut_rotSpeed_info : Outport  Port=17
  hvs_zfCetrax_gbxOut_Acc_info : Outport  Port=18
  hvs_zfCetrax_gbx_gearRatio_tgt_info : Outport  Port=19
  hvs_zfCetrax_gbx_emDec_active_info : Outport  Port=20
  hvs_zfCetrax_gbx_pwrLoss_info : Outport  Port=21
  hvs_zfCetrax_derating_active_info : Outport  Port=22
  hvs_zfCetrax_gbx_gearRatio : Outport  Port=23
  hvs_zfCetrax_gbxOut_rotSpeed : Outport  Port=24
  hvs_zfCetrax_gbx_gearShift_active : Outport  Port=25
  hvs_zfCetrax_pe1_curDC : Outport  Port=26
  hvs_zfCetrax_pe2_curDC : Outport  Port=27
  hvs_zfCetrax_drv_drivingState_info : Outport  Port=28
  wires:
  MotorSelection/1(Emot1_Selection) -> [Emot1_Selection]
  MotorSelection/2(Emot2_Selection) -> [Emot2_Selection]
  MotorSelection/3(Emot3_Selection) -> [Emot3_Selection]
  MotorSelection/4(Emot4_Selection) -> [Emot4_Selection]
  [Emot1_Selection] -> Emot1_4/4(Emot1_Selection)
  voltBatHV1/1 -> [voltBat], Emot1_4/1(voltBatHV1)
  pti_EMD1_TrqReq_Nm/1 -> EMD1_Selection/1(pti_EMD1_TrqReq_Nm)
  pti_EMD1_ControlMode/1 -> EMD1_Selection/2(pti_EMD1_ControlMode)
  edcu_EMD1_CMD_TorqueRefLim/1 -> EMD1_Selection/3(edcu_EMD1_CMD_TorqueRefLim)
  edcu_EMD1_CMD_ControlMode/1 -> EMD1_Selection/4(edcu_EMD1_CMD_ControlMode)
  EMD1_Selection/1(Signal) -> Bus Selector/1
  Bus Selector/1 -> Emot1_4/2(trqEmotDesPhy1)  "<EMD1_TrqReq_Nm>"
  Bus Selector/2 -> Emot1_4/3(emot_CMD1)  "<EMD1_ControlMode>"
  drv_AccPdl_pos/1 -> Emot1_4/5(drv_AccPdl_pos)
  drv_BrkPdl_pos/1 -> Emot1_4/6(drv_BrkPdl_pos)
  env_Temperature/1 -> Emot1_4/7(env_Temperature)
  env_road_slope_pct/1 -> Emot1_4/8(env_road_slope_pct)
  drv_HaltBrkSw_Rq/1 -> Emot1_4/9(drv_HaltBrkSw_Rq)
  hvs_veh_GenericLoss_transVel/1 -> Emot1_4/10(veh_linVel)
  pti_zfCetrax_ctrl_em_pwrElec_min/1 -> Emot1_4/15(em_pwrElec_min)
  drv_v_des_max_kmh/1 -> Emot1_4/11(veh_linVel_tgt)
  hvs_veh_GenericLoss_transAcc/1 -> Emot1_4/12(veh_linAcc)
  pti_zfCetrax_ctrl_em_pwrElec_max/1 -> Emot1_4/16(em_pwrElec_max)
  hvs_zfCetrax_gbxOut_resTrq/1 -> Emot1_4/13(veh_resTrq_gbxOut)
  hvs_zfCetrax_gbxOut_veh_inertia/1 -> Emot1_4/14(veh_inertial_gbxOut)
  Emot1_4/1(ceTrax) -> Bus Selector4/1, Bus Selector3/1, Bus Selector2/1, Bus Selector13/1, Bus Selector8/1, Bus Selector7/1, Bus Selector1/1
  Bus Selector1/1 -> hvs_zfCetrax_gbxOut_torque/1  "<gbxOut_trq>"
  Bus Selector4/1 -> Add/1, [pe1_curDC]  "<pe1_curDC>"
  Bus Selector4/2 -> [pe2_curDC], Add/2  "<pe2_curDC>"
  Add/1 -> hvs_dcLink_drive_emot_current/1
  Bus Selector7/1 -> Add1/1  "<em1_pwrLoss>"
  Bus Selector7/2 -> Add1/2  "<em2_pwrLoss>"
  Add1/1 -> watt2kW/1
  Bus Selector8/2 -> Product/2  "<em1_rotSpeed>"
  Bus Selector8/1 -> [em1_trq], Product/1  "<em1_trq>"
  Product/1 -> Add2/1
  Bus Selector8/3 -> Add2/2  "<em1_pwrLoss>"
  Add2/1 -> Add4/1
  Bus Selector13/1 -> [em2_trq], Product1/1  "<em2_trq>"
  Bus Selector13/2 -> Product1/2  "<em2_rotSpeed>"
  Product1/1 -> Add3/1
  Bus Selector13/3 -> Add3/2  "<em2_pwrLoss>"
  Add3/1 -> Add5/1
  [pe1_curDC] -> Product2/2
  Product2/1 -> Add4/2
  [voltBat] -> Product2/1
  [pe2_curDC] -> Product3/2
  Product3/1 -> Add5/2
  [voltBat] -> Product3/1
  Add4/1 -> Add6/1
  Add5/1 -> Add6/2
  Add6/1 -> watt2kW1/1
  watt2kW/1 -> hvs_drvEmotWasteHeat_power/1, [zfCetrax_drvEmotWasteHear_power]
  watt2kW1/1 -> hvs_driveInverterWasteHeat_power/1, [zfCetrax_driveInverterWasteHeat_power]
  [voltBat] -> hvs_zfCetrax_drive_emot_voltage/1
  Bus Selector2/1 -> hvs_zfCetrax_gbx_gearAct/1  "<gbx_gearAct>"
  Bus Selector2/5 -> hvs_zfCetrax_em1_trqPotential_min/1  "<em1_trqPotential_min>"
  Bus Selector2/6 -> hvs_zfCetrax_em1_trqPotential_max/1  "<em1_trqPotential_max>"
  Bus Selector2/7 -> hvs_zfCetrax_em2_trqPotential_min/1  "<em2_trqPotential_min>"
  Bus Selector2/8 -> hvs_zfCetrax_em2_trqPotential_max/1  "<em2_trqPotential_max>"
  Bus Selector2/10 -> hvs_zfCetrax_em2_rotSpeed/1  "<em2_rotSpeed>"
  Bus Selector2/9 -> hvs_zfCetrax_em1_rotSpeed/1  "<em1_rotSpeed>"
  [zfCetrax_drvEmotWasteHear_power] -> Gain/1
  Gain/1 -> hvs_zfCetrax_drvEmotWasteHeat_power/1
  [zfCetrax_driveInverterWasteHeat_power] -> Gain1/1
  Gain1/1 -> hvs_zfCetrax_driveInverterWasteHeat_power/1
  [em1_trq] -> Gain2/1
  [em2_trq] -> Gain3/1
  Gain2/1 -> hvs_zfCetrax_em1_trq/1
  Gain3/1 -> hvs_zfCetrax_em2_trq/1
  pti_WheelBrake_trq/1 -> Manual Switch/1
  Bus Selector3/1 -> hvs_zfCetrax_gbxOut_rotSpeed_info/1  "<gbxOut_rotSpeed>"
  Bus Selector3/2 -> hvs_zfCetrax_gbxOut_Acc_info/1  "<gbxOut_Acc>"
  Bus Selector3/3 -> hvs_zfCetrax_gbx_gearRatio_tgt_info/1  "<gbx_gearRatio_tgt>"
  Bus Selector3/4 -> hvs_zfCetrax_gbx_emDec_active_info/1  "<gbx_emDec_active>"
  Bus Selector3/5 -> hvs_zfCetrax_gbx_pwrLoss_info/1  "<gbx_pwrLoss>"
  Bus Selector3/6 -> hvs_zfCetrax_derating_active_info/1  "<derating_active>"
  Bus Selector2/2 -> Gain4/1  "<gbx_gearRatio_tgt>"
  Gain4/1 -> hvs_zfCetrax_gbx_gearRatio/1
  hvs_zfCetrax_vehWheel_brk_torque/1 -> Manual Switch/2
  Manual Switch/1 -> Emot1_4/17(pti_WheelBrake_trq)
  Bus Selector2/4 -> hvs_zfCetrax_gbxOut_rotSpeed/1  "<gbxOut_rotSpeed>"
  Bus Selector2/3 -> hvs_zfCetrax_gbx_gearShift_active/1  "<gbx_gearShift_active>"
  Bus Selector2/11 -> hvs_zfCetrax_pe1_curDC/1  "<pe1_curDC>"
  Bus Selector2/12 -> hvs_zfCetrax_pe2_curDC/1  "<pe2_curDC>"
  Bus Selector3/7 -> hvs_zfCetrax_drv_drivingState_info/1  "<drv_drivingState>"

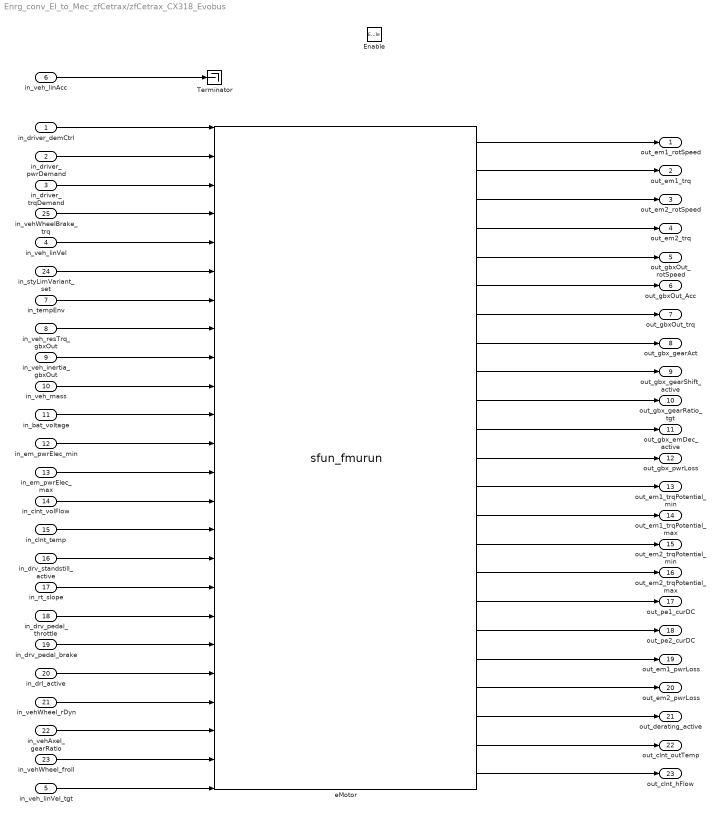
== system Enrg_conv_El_to_Mec_zfCetrax/zfCetrax_CX318_Evobus ==
  in_driver_demCtrl : Inport
  in_driver_pwrDemand : Inport  Port=2
  in_driver_trqDemand : Inport  Port=3
  in_veh_linVel : Inport  Port=4
  in_veh_linVel_tgt : Inport  Port=5
  in_veh_linAcc : Inport  Port=6
  in_tempEnv : Inport  Port=7
  in_veh_resTrq_gbxOut : Inport  Port=8
  in_veh_inertia_gbxOut : Inport  Port=9
  in_veh_mass : Inport  Port=10
  in_bat_voltage : Inport  Port=11
  in_em_pwrElec_min : Inport  Port=12
  in_em_pwrElec_max : Inport  Port=13
  in_clnt_volFlow : Inport  Port=14
  in_clnt_temp : Inport  Port=15
  in_drv_standstill_active : Inport  Port=16
  in_rt_slope : Inport  Port=17
  in_drv_pedal_throttle : Inport  Port=18
  in_drv_pedal_brake : Inport  Port=19
  in_drl_active : Inport  Port=20
  in_vehWheel_rDyn : Inport  Port=21
  in_vehAxel_gearRatio : Inport  Port=22
  in_vehWheel_froll : Inport  Port=23
  in_styLimVariant_set : Inport  Port=24
  in_vehWheelBrake_trq : Inport  Port=25
  Enable : EnablePort
  Terminator : Terminator
  eMotor : S-Function  LoadFcn=FMIKit.setSFunctionParameters(gcb)  FunctionName=sfun_fmurun  Parameters='2.0' 1 '{6df466fc-55df-48cc-82e1-ee408b9f2dc3}' 'CustomerVar1_Master' FMIKit.getUnzipDirectory(gcb) 0 0 0 '' 0 -1 0 0 0 [] [] [] [] char({}) [1 1 1 1 1 1 1 1 1 1 1 1 1 1 1 1 1 1 1 1 1 1 1 1] [0 0 0 0 0 0 0 0 0 0 0 0 0 0 0 0 0 0 0 0 0 0 0 0] [0 0 0 0 0 0 0 0 0 0 0 0 0 0 0 0 0 0 0 0 0 0 0 0] [1 2 3 4 5 6 7 8 9 10 11 12 13 14 15 16 17 18 19 20 21 22 23 24] [1 1 1 1 1 1 1 1 1 1 1 1 1 1 1 1 1 1 1 1 1 1 1] [0 0 0 0 0 0 0 0 2 0 0 0 0 0 0 0 0 0 0 0 0 0 0] [25 26 27 28 29 30 31 32 33 34 35 36 37 38 39 40 41 42 43 44 45 46 47]  SFunctionDeploymentMode=off  EnableBusSupport=off
      settings: DeleteFcn=FMIKit.closeBlockDialog(gcbh)  ModelCloseFcn=FMIKit.closeBlockDialog(gcbh)  DestroyFcn=FMIKit.closeBlockDialog(gcbh)  OpenFcn=FMIKit.showBlockDialog(gcbh);  CloseFcn=FMIKit.closeBlockDialog(gcbh)  ParentCloseFcn=FMIKit.closeBlockDialog(gcbh)
      mask Help: eval('FMIKit.showBlockDialogHelp();')
      mask Display:
      | ports = get_param(gcb, 'Ports');
      | 
      | inports = FMIKit.getInportLabels(gcb);
      | 
      | for i = 1:min(numel(inports), ports(1))
      |     port_label('input', i, inports{i})
      | end
      | 
      | outports = FMIKit.getOutportLabels(gcb);
      | 
      | for i = 1:min(numel(outports), ports(2))
      |     port_label('output', i, outports{i})
      | end
      | 
      | if isempty(inports) && isempty(outports)
      |     patch([-20 65, 65 -20], [-20 -20 70 70], [1 1 1])
      |     plot([-2 50 50 -2 -2], [0 0 50 50 0])
      |     patch([-9 12 12 -9 -9], [12 12 20 20 12], [1 1 1])
      |     plot([-9 12 12 -9 -9], [12 12 20 20 12])
      |     patch([-9 12 12 -9 -9], [30 30 38 38 30], [1 1 1])
      |     plot([-9 12 12 -9 -9], [30 30 38 38 30])
      | end
  out_em1_rotSpeed : Outport
  out_em1_trq : Outport  Port=2
  out_em2_rotSpeed : Outport  Port=3
  out_em2_trq : Outport  Port=4
  out_gbxOut_rotSpeed : Outport  Port=5
  out_gbxOut_Acc : Outport  Port=6
  out_gbxOut_trq : Outport  Port=7
  out_gbx_gearAct : Outport  Port=8
  out_gbx_gearShift_active : Outport  Port=9
  out_gbx_gearRatio_tgt : Outport  Port=10
  out_gbx_emDec_active : Outport  Port=11
  out_gbx_pwrLoss : Outport  Port=12
  out_em1_trqPotential_min : Outport  Port=13
  out_em1_trqPotential_max : Outport  Port=14
  out_em2_trqPotential_min : Outport  Port=15
  out_em2_trqPotential_max : Outport  Port=16
  out_pe1_curDC : Outport  Port=17
  out_pe2_curDC : Outport  Port=18
  out_em1_pwrLoss : Outport  Port=19
  out_em2_pwrLoss : Outport  Port=20
  out_derating_active : Outport  Port=21
  out_clnt_outTemp : Outport  Port=22
  out_clnt_hFlow : Outport  Port=23
  wires:
  in_vehWheel_froll/1 -> eMotor/23
  in_vehAxel_gearRatio/1 -> eMotor/22
  in_vehWheel_rDyn/1 -> eMotor/21
  in_driver_demCtrl/1 -> eMotor/1
  in_driver_trqDemand/1 -> eMotor/3
  in_veh_linVel/1 -> eMotor/5
  in_veh_linVel_tgt/1 -> eMotor/24
  in_tempEnv/1 -> eMotor/7
  in_veh_resTrq_gbxOut/1 -> eMotor/8
  in_veh_inertia_gbxOut/1 -> eMotor/9
  in_veh_mass/1 -> eMotor/10
  in_bat_voltage/1 -> eMotor/11
  in_em_pwrElec_min/1 -> eMotor/12
  in_em_pwrElec_max/1 -> eMotor/13
  in_clnt_volFlow/1 -> eMotor/14
  in_clnt_temp/1 -> eMotor/15
  in_drv_standstill_active/1 -> eMotor/16
  in_rt_slope/1 -> eMotor/17
  in_drv_pedal_throttle/1 -> eMotor/18
  in_drv_pedal_brake/1 -> eMotor/19
  in_drl_active/1 -> eMotor/20
  in_driver_pwrDemand/1 -> eMotor/2
  in_veh_linAcc/1 -> Terminator/1
  eMotor/1 -> out_em1_rotSpeed/1
  eMotor/2 -> out_em1_trq/1
  eMotor/3 -> out_em2_rotSpeed/1
  eMotor/4 -> out_em2_trq/1
  eMotor/5 -> out_gbxOut_rotSpeed/1
  eMotor/6 -> out_gbxOut_Acc/1
  eMotor/7 -> out_gbxOut_trq/1
  eMotor/8 -> out_gbx_gearAct/1
  eMotor/9 -> out_gbx_gearShift_active/1
  eMotor/10 -> out_gbx_gearRatio_tgt/1
  eMotor/11 -> out_gbx_emDec_active/1
  eMotor/12 -> out_gbx_pwrLoss/1
  eMotor/13 -> out_em1_trqPotential_min/1
  eMotor/14 -> out_em1_trqPotential_max/1
  eMotor/15 -> out_em2_trqPotential_min/1
  eMotor/16 -> out_em2_trqPotential_max/1
  eMotor/17 -> out_pe1_curDC/1
  eMotor/18 -> out_pe2_curDC/1
  eMotor/19 -> out_em1_pwrLoss/1
  eMotor/20 -> out_em2_pwrLoss/1
  eMotor/21 -> out_derating_active/1
  eMotor/22 -> out_clnt_outTemp/1
  eMotor/23 -> out_clnt_hFlow/1
  in_styLimVariant_set/1 -> eMotor/6
  in_vehWheelBrake_trq/1 -> eMotor/4

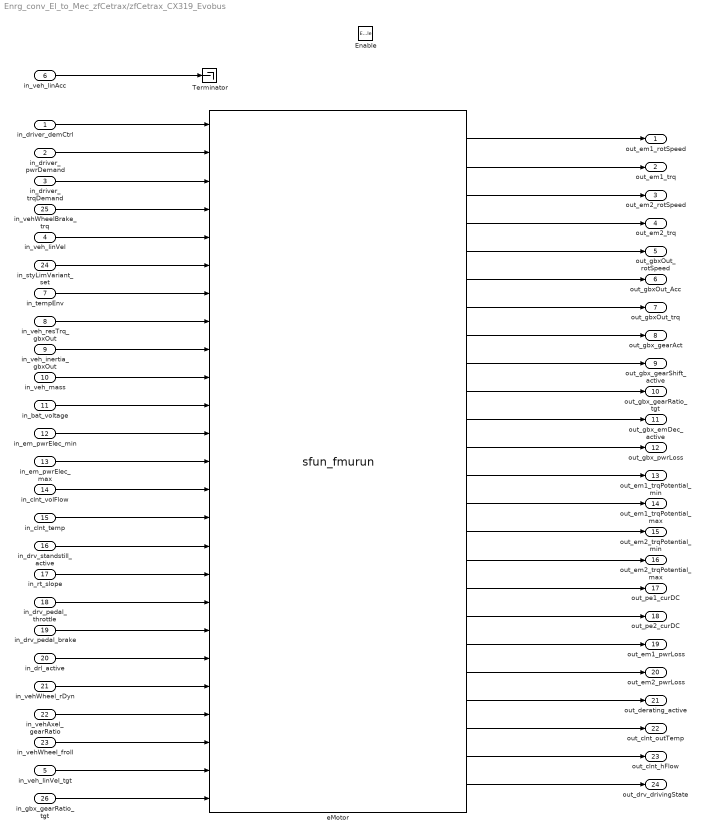
== system Enrg_conv_El_to_Mec_zfCetrax/zfCetrax_CX319_Evobus ==
  in_driver_demCtrl : Inport
  in_driver_pwrDemand : Inport  Port=2
  in_driver_trqDemand : Inport  Port=3
  in_veh_linVel : Inport  Port=4
  in_veh_linVel_tgt : Inport  Port=5
  in_veh_linAcc : Inport  Port=6
  in_tempEnv : Inport  Port=7
  in_veh_resTrq_gbxOut : Inport  Port=8
  in_veh_inertia_gbxOut : Inport  Port=9
  in_veh_mass : Inport  Port=10
  in_bat_voltage : Inport  Port=11
  in_em_pwrElec_min : Inport  Port=12
  in_em_pwrElec_max : Inport  Port=13
  in_clnt_volFlow : Inport  Port=14
  in_clnt_temp : Inport  Port=15
  in_drv_standstill_active : Inport  Port=16
  in_rt_slope : Inport  Port=17
  in_drv_pedal_throttle : Inport  Port=18
  in_drv_pedal_brake : Inport  Port=19
  in_drl_active : Inport  Port=20
  in_vehWheel_rDyn : Inport  Port=21
  in_vehAxel_gearRatio : Inport  Port=22
  in_vehWheel_froll : Inport  Port=23
  in_styLimVariant_set : Inport  Port=24
  in_vehWheelBrake_trq : Inport  Port=25
  in_gbx_gearRatio_tgt : Inport  Port=26
  Enable : EnablePort
  Terminator : Terminator
  eMotor : S-Function  LoadFcn=FMIKit.setSFunctionParameters(gcb)  FunctionName=sfun_fmurun  Parameters='2.0' 1 '{87150a17-60fe-aceb-d5f0-c416d2a9791d}' 'CustomerVar_EvoBusCX319' FMIKit.getUnzipDirectory(gcb) 0 0 0 '' 0 -1 0 0 0 [] [] [] [] char({}) [1 1 1 1 1 1 1 1 1 1 1 1 1 1 1 1 1 1 1 1 1 1 1 1 1] [0 0 0 0 0 0 0 0 0 0 0 0 0 0 0 0 0 0 0 0 0 0 0 0 0] [0 0 0 0 0 0 0 0 0 0 0 0 0 0 0 0 0 0 0 0 0 0 0 0 0] [0 1 2 3 4 5 6 7 8 9 10 11 12 13 14 15 16 17 18 19 20 21 22 23 24] [1 1 1 1 1 1 1 1 1 1 1 1 1 1 1 1 1 1 1 1 1 1 1 1] [0 0 0 0 0 0 0 0 0 0 0 0 0 0 0 0 0 0 0 0 0 0 0 0] [25 26 27 28 29 30 31 32 33 34 35 36 37 38 39 40 41 42 43 44 45 46 47 48]  SFunctionDeploymentMode=off  EnableBusSupport=off
      settings: DeleteFcn=FMIKit.closeBlockDialog(gcbh)  ModelCloseFcn=FMIKit.closeBlockDialog(gcbh)  DestroyFcn=FMIKit.closeBlockDialog(gcbh)  OpenFcn=FMIKit.showBlockDialog(gcbh);  CloseFcn=FMIKit.closeBlockDialog(gcbh)  ParentCloseFcn=FMIKit.closeBlockDialog(gcbh)
      mask Help: eval('FMIKit.showBlockDialogHelp();')
      mask Display:
      | ports = get_param(gcb, 'Ports');
      | 
      | inports = FMIKit.getInportLabels(gcb);
      | 
      | for i = 1:min(numel(inports), ports(1))
      |     port_label('input', i, inports{i})
      | end
      | 
      | outports = FMIKit.getOutportLabels(gcb);
      | 
      | for i = 1:min(numel(outports), ports(2))
      |     port_label('output', i, outports{i})
      | end
      | 
      | if isempty(inports) && isempty(outports)
      |     patch([-20 65, 65 -20], [-20 -20 70 70], [1 1 1])
      |     plot([-2 50 50 -2 -2], [0 0 50 50 0])
      |     patch([-9 12 12 -9 -9], [12 12 20 20 12], [1 1 1])
      |     plot([-9 12 12 -9 -9], [12 12 20 20 12])
      |     patch([-9 12 12 -9 -9], [30 30 38 38 30], [1 1 1])
      |     plot([-9 12 12 -9 -9], [30 30 38 38 30])
      | end
  out_em1_rotSpeed : Outport
  out_em1_trq : Outport  Port=2
  out_em2_rotSpeed : Outport  Port=3
  out_em2_trq : Outport  Port=4
  out_gbxOut_rotSpeed : Outport  Port=5
  out_gbxOut_Acc : Outport  Port=6
  out_gbxOut_trq : Outport  Port=7
  out_gbx_gearAct : Outport  Port=8
  out_gbx_gearShift_active : Outport  Port=9
  out_gbx_gearRatio_tgt : Outport  Port=10
  out_gbx_emDec_active : Outport  Port=11
  out_gbx_pwrLoss : Outport  Port=12
  out_em1_trqPotential_min : Outport  Port=13
  out_em1_trqPotential_max : Outport  Port=14
  out_em2_trqPotential_min : Outport  Port=15
  out_em2_trqPotential_max : Outport  Port=16
  out_pe1_curDC : Outport  Port=17
  out_pe2_curDC : Outport  Port=18
  out_em1_pwrLoss : Outport  Port=19
  out_em2_pwrLoss : Outport  Port=20
  out_derating_active : Outport  Port=21
  out_clnt_outTemp : Outport  Port=22
  out_clnt_hFlow : Outport  Port=23
  out_drv_drivingState : Outport  Port=24
  wires:
  in_vehWheelBrake_trq/1 -> eMotor/4
  in_styLimVariant_set/1 -> eMotor/6
  eMotor/23 -> out_clnt_hFlow/1
  eMotor/22 -> out_clnt_outTemp/1
  eMotor/21 -> out_derating_active/1
  eMotor/20 -> out_em2_pwrLoss/1
  eMotor/19 -> out_em1_pwrLoss/1
  eMotor/18 -> out_pe2_curDC/1
  eMotor/17 -> out_pe1_curDC/1
  eMotor/16 -> out_em2_trqPotential_max/1
  eMotor/15 -> out_em2_trqPotential_min/1
  eMotor/14 -> out_em1_trqPotential_max/1
  eMotor/13 -> out_em1_trqPotential_min/1
  eMotor/12 -> out_gbx_pwrLoss/1
  eMotor/11 -> out_gbx_emDec_active/1
  eMotor/10 -> out_gbx_gearRatio_tgt/1
  eMotor/9 -> out_gbx_gearShift_active/1
  eMotor/8 -> out_gbx_gearAct/1
  eMotor/7 -> out_gbxOut_trq/1
  eMotor/6 -> out_gbxOut_Acc/1
  eMotor/5 -> out_gbxOut_rotSpeed/1
  eMotor/4 -> out_em2_trq/1
  eMotor/3 -> out_em2_rotSpeed/1
  eMotor/2 -> out_em1_trq/1
  eMotor/1 -> out_em1_rotSpeed/1
  in_veh_linAcc/1 -> Terminator/1
  in_driver_pwrDemand/1 -> eMotor/2
  in_drl_active/1 -> eMotor/20
  in_drv_pedal_brake/1 -> eMotor/19
  in_drv_pedal_throttle/1 -> eMotor/18
  in_rt_slope/1 -> eMotor/17
  in_drv_standstill_active/1 -> eMotor/16
  in_clnt_temp/1 -> eMotor/15
  in_clnt_volFlow/1 -> eMotor/14
  in_em_pwrElec_max/1 -> eMotor/13
  in_em_pwrElec_min/1 -> eMotor/12
  in_bat_voltage/1 -> eMotor/11
  in_veh_mass/1 -> eMotor/10
  in_veh_inertia_gbxOut/1 -> eMotor/9
  in_veh_resTrq_gbxOut/1 -> eMotor/8
  in_tempEnv/1 -> eMotor/7
  in_veh_linVel_tgt/1 -> eMotor/24
  in_veh_linVel/1 -> eMotor/5
  in_driver_trqDemand/1 -> eMotor/3
  in_driver_demCtrl/1 -> eMotor/1
  in_vehWheel_rDyn/1 -> eMotor/21
  in_vehAxel_gearRatio/1 -> eMotor/22
  in_vehWheel_froll/1 -> eMotor/23
  in_gbx_gearRatio_tgt/1 -> eMotor/25
  eMotor/24 -> out_drv_drivingState/1
